simulink model "PI_IP_SimulationComparison"  (R2018a)
settings: Solver=FixedStepAuto  StartTime=0.0  StopTime=20  RelTol=1e-3
PreLoadFcn:
  | % plant
  | K0=0.82;
  | tau0=0.26;
  | 
  | % Sampling time
  | Ts=0.01;
  | 
  | % Especifications
  | xi=1;
  | ts_2=0.8; % settling time with %2 criterion
  | Tdes=ts_2/4;
  | wn=5.8/(xi*ts_2);
  | 
  | % Controller design
  | Zdes=exp(-Ts/Tdes);
  | alpha=exp(-Ts/tau0);
  | beta=-2*exp(-Ts*xi*wn)*cos(wn*Ts*sqrt(1-xi^2));
  | gamma=exp(-2*Ts*xi*wn);
  | 
  | Ki_star=(gamma-alpha+beta+(alpha+1))/(2*K0*(1-alpha));
  | Ki=(2/Ts)*Ki_star;
  | Kp=((beta+alpha+1)/(K0*(1-alpha)))-Ki_star;
values from neighbouring files (symbols this model uses):
  Kaw = 1/Ki    [PI_sinto.m]
undefined symbols (not defined in the file or in its folder): DiscIntNeverNeededParam
libraries: simulink x3
settings Model: ExtModeTrigDuration=2  Creator=Eneko Lerma  LastModifiedBy=Eneko Lerma
settings OptimizationCC: EnhancedBackFolding=on  PassReuseOutputArgsAs=Individual arguments  MaxStackSize=64  OptimizeBlockOrder=speed  DifferentSizesBufferReuse=on  OptimizationCustomize=off
settings DebuggingCC: ParameterPrecisionLossMsg=none  ParameterTunabilityLossMsg=error
settings HardwareCC: ProdBitPerPointer=32  ProdBitPerSizeT=32  ProdBitPerPtrDiffT=32  ProdLargestAtomicInteger=Long  ProdLargestAtomicFloat=Double  ProdWordSize=32  ProdHWDeviceType=ARM Compatible->ARM Cortex
settings SFSimCC: MATLABDynamicMemAlloc=off
settings RTWCC: SystemTargetFile=ert.tlc  HardwareBoard=Arduino Due  TLCOptions=-aInlineSetEventsForThisBaseRateFcn=TLC_FALSE -aSuppressMultiTaskScheduler=TLC_FALSE -aRateBasedStepFcn=1  TemplateMakefile=ert_default_tmf  GenerateReport=on  Toolchain=Arduino ARM  BuildConfiguration=Faster Runs  IncludeHyperlinkInReport=on  LaunchReport=on  GenerateTraceInfo=on  GenerateTraceReport=on  GenerateTraceReportSl=on  GenerateTraceReportSf=on  GenerateTraceReportEml=on
settings CodeAppCC: ForceParamTrailComments=on  IgnoreCustomStorageClasses=off  OperatorAnnotations=on  SimulinkDataObjDesc=on  SFDataObjDesc=on  InsertBlockDesc=on
settings ERTTargetCC: SupportContinuousTime=on  SupportVariableSizeSignals=on

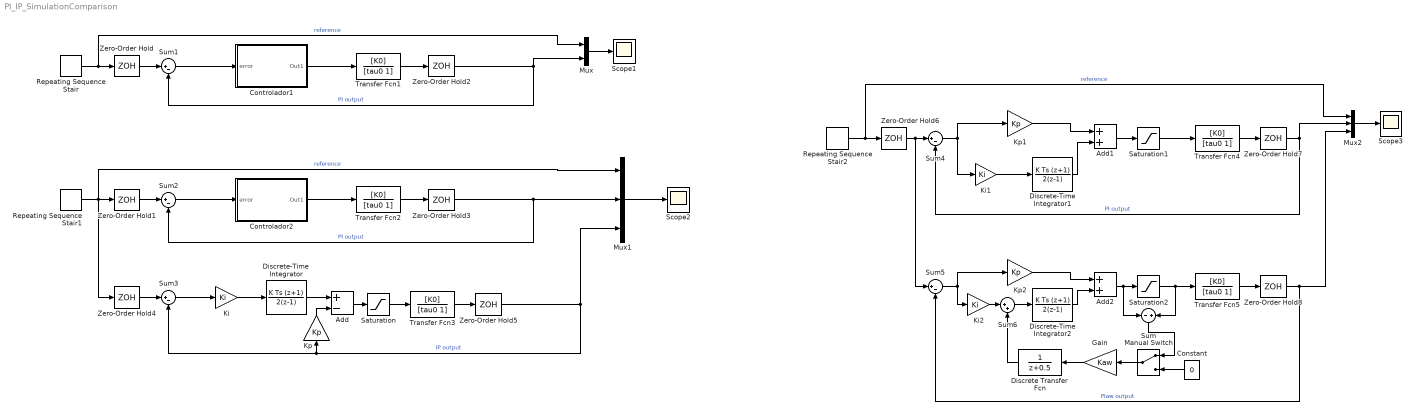
== system PI_IP_SimulationComparison ==
  Add : Sum  Inputs=+-  AccumDataTypeStr=single
  Add1 : Sum  AccumDataTypeStr=single
  Add2 : Sum  AccumDataTypeStr=single
  Constant : Constant  Value=0  SampleTime=Ts
  Controlador1 : Subsystem
  Controlador2 : Subsystem
  Discrete Transfer Fcn : DiscreteTransferFcn  SampleTime=Ts
  Discrete-Time Integrator : DiscreteIntegrator  IntegratorMethod=Integration: Trapezoidal  SampleTime=Ts  OutDataTypeStr=single  ICPrevOutput=DiscIntNeverNeededParam  ICPrevScaledInput=DiscIntNeverNeededParam
  Discrete-Time Integrator1 : DiscreteIntegrator  IntegratorMethod=Integration: Trapezoidal  SampleTime=Ts  OutDataTypeStr=single  ICPrevOutput=DiscIntNeverNeededParam  ICPrevScaledInput=DiscIntNeverNeededParam
  Discrete-Time Integrator2 : DiscreteIntegrator  IntegratorMethod=Integration: Trapezoidal  SampleTime=Ts  OutDataTypeStr=single  ICPrevOutput=DiscIntNeverNeededParam  ICPrevScaledInput=DiscIntNeverNeededParam
  Gain : Gain  Gain=Kaw
  Ki : Gain  Gain=Ki
  Ki1 : Gain  Gain=Ki
  Ki2 : Gain  Gain=Ki
  Kp : Gain  Gain=Kp  OutDataTypeStr=single
  Kp1 : Gain  Gain=Kp  OutDataTypeStr=single
  Kp2 : Gain  Gain=Kp  OutDataTypeStr=single
  Manual Switch : ManualSwitch
  Mux : Mux  Inputs=2
  Mux1 : Mux  Inputs=3
  Mux2 : Mux  Inputs=3
  Repeating Sequence Stair : simulink/Sources/Repeating Sequence Stair  OutValues=[0 2 -2 -1].'  tsamp=4  OutMin=[]  OutMax=[]  OutDataTypeStr=double  OutputDataTypeScalingMode=double  OutDataType=fixdt(0,8)  ConRadixGroup=Best Precision: Vector-wise  OutScaling=2^-12
  Repeating Sequence Stair1 : simulink/Sources/Repeating Sequence Stair  OutValues=[0 2 -2 -1].'  tsamp=4  OutMin=[]  OutMax=[]  OutDataTypeStr=double  OutputDataTypeScalingMode=double  OutDataType=fixdt(0,8)  ConRadixGroup=Best Precision: Vector-wise  OutScaling=2^-12
  Repeating Sequence Stair2 : simulink/Sources/Repeating Sequence Stair  OutValues=[0 2 -2 -1].'  tsamp=4  OutMin=[]  OutMax=[]  OutDataTypeStr=double  OutputDataTypeScalingMode=double  OutDataType=fixdt(0,8)  ConRadixGroup=Best Precision: Vector-wise  OutScaling=2^-12
  Saturation : Saturate  UpperLimit=5  LowerLimit=-5  OutDataTypeStr=double
  Saturation1 : Saturate  UpperLimit=5  LowerLimit=-5  OutDataTypeStr=double
  Saturation2 : Saturate  UpperLimit=5  LowerLimit=-5  OutDataTypeStr=double
  Scope1 : Scope
  Scope2 : Scope
  Scope3 : Scope
  Sum : Sum  Inputs=-|+
  Sum{1..5} (5 alike) : Sum  Inputs=|+-  AccumDataTypeStr=single
  Sum6 : Sum  Inputs=|++
  Transfer Fcn{1..5} (5 alike) : TransferFcn  Numerator=[K0]  Denominator=[tau0 1]
  Zero-Order Hold{,1..8} (9 alike) : ZeroOrderHold  SampleTime=Ts
  wires:
  Zero-Order Hold/1 -> Sum1/1
  Controlador1/1(Out1) -> Transfer Fcn1/1
  Sum1/1 -> Controlador1/1(error)
  Transfer Fcn1/1 -> Zero-Order Hold2/1
  Zero-Order Hold2/1 -> Mux/2, Sum1/2  "PI output"
  Mux/1 -> Scope1/1
  Repeating Sequence Stair/1 -> Mux/1, Zero-Order Hold/1  "reference"
  Mux1/1 -> Scope2/1
  Zero-Order Hold1/1 -> Sum2/1
  Repeating Sequence Stair1/1 -> Zero-Order Hold4/1, Mux1/1, Zero-Order Hold1/1  "reference"
  Zero-Order Hold3/1 -> Sum2/2, Mux1/2  "PI output"
  Sum2/1 -> Controlador2/1(error)
  Transfer Fcn2/1 -> Zero-Order Hold3/1
  Controlador2/1(Out1) -> Transfer Fcn2/1
  Transfer Fcn3/1 -> Zero-Order Hold5/1
  Zero-Order Hold5/1 -> Mux1/3, Kp/1, Sum3/2  "IP output"
  Zero-Order Hold4/1 -> Sum3/1
  Sum3/1 -> Ki/1
  Ki/1 -> Discrete-Time Integrator/1
  Saturation/1 -> Transfer Fcn3/1
  Kp/1 -> Add/2
  Discrete-Time Integrator/1 -> Add/1
  Add/1 -> Saturation/1
  Zero-Order Hold7/1 -> Mux2/2, Sum4/2  "PI output"
  Mux2/1 -> Scope3/1
  Repeating Sequence Stair2/1 -> Mux2/1, Zero-Order Hold6/1  "reference"
  Saturation1/1 -> Transfer Fcn4/1
  Transfer Fcn4/1 -> Zero-Order Hold7/1
  Zero-Order Hold6/1 -> Sum5/1, Sum4/1
  Add1/1 -> Saturation1/1
  Sum4/1 -> Ki1/1, Kp1/1
  Discrete-Time Integrator1/1 -> Add1/2
  Kp1/1 -> Add1/1
  Ki1/1 -> Discrete-Time Integrator1/1
  Sum5/1 -> Ki2/1, Kp2/1
  Ki2/1 -> Sum6/1
  Kp2/1 -> Add2/1
  Discrete-Time Integrator2/1 -> Add2/2
  Transfer Fcn5/1 -> Zero-Order Hold8/1
  Zero-Order Hold8/1 -> Mux2/3, Sum5/2  "PIaw output"
  Manual Switch/1 -> Gain/1
  Add2/1 -> Sum/1, Saturation2/1
  Constant/1 -> Manual Switch/2
  Saturation2/1 -> Sum/2, Transfer Fcn5/1
  Sum/1 -> Manual Switch/1
  Gain/1 -> Discrete Transfer Fcn/1
  Sum6/1 -> Discrete-Time Integrator2/1
  Discrete Transfer Fcn/1 -> Sum6/2

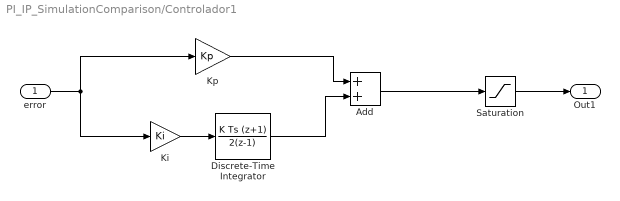
== system PI_IP_SimulationComparison/Controlador1 ==
  error : Inport
  Add : Sum  AccumDataTypeStr=single
  Discrete-Time Integrator : DiscreteIntegrator  IntegratorMethod=Integration: Trapezoidal  SampleTime=Ts  OutDataTypeStr=single  ICPrevOutput=DiscIntNeverNeededParam  ICPrevScaledInput=DiscIntNeverNeededParam
  Ki : Gain  Gain=Ki
  Kp : Gain  Gain=Kp  OutDataTypeStr=single
  Saturation : Saturate  UpperLimit=5  LowerLimit=-5  OutDataTypeStr=double
  Out1 : Outport  OutDataTypeStr=double
  wires:
  error/1 -> Kp/1, Ki/1
  Saturation/1 -> Out1/1
  Add/1 -> Saturation/1
  Ki/1 -> Discrete-Time Integrator/1
  Discrete-Time Integrator/1 -> Add/2
  Kp/1 -> Add/1

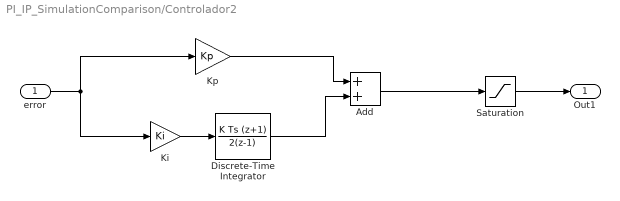
== system PI_IP_SimulationComparison/Controlador2 ==
  error : Inport
  Add : Sum  AccumDataTypeStr=single
  Discrete-Time Integrator : DiscreteIntegrator  IntegratorMethod=Integration: Trapezoidal  SampleTime=Ts  OutDataTypeStr=single  ICPrevOutput=DiscIntNeverNeededParam  ICPrevScaledInput=DiscIntNeverNeededParam
  Ki : Gain  Gain=Ki
  Kp : Gain  Gain=Kp  OutDataTypeStr=single
  Saturation : Saturate  UpperLimit=5  LowerLimit=-5  OutDataTypeStr=double
  Out1 : Outport  OutDataTypeStr=double
  wires:
  error/1 -> Kp/1, Ki/1
  Saturation/1 -> Out1/1
  Add/1 -> Saturation/1
  Ki/1 -> Discrete-Time Integrator/1
  Discrete-Time Integrator/1 -> Add/2
  Kp/1 -> Add/1
